simulink model "AD_SOAR_c7_V2f_c73_Clean_original"  (R2021a)
settings: Solver=ode4  StartTime=0.0  StopTime=TMax  FixedStep=Control.DT  RelTol=1e-3
undefined symbols (not defined in the file): Control, DiscIntNeverNeededParam, dLPF_slow, Downratelimiter, DT, IPCDQ_LPF, LPF_SetSmooth, OLControlParams, OutList, Parameters, PitchControlParams, rpm2radps, S_LowBPLim, Simulation, strmatch, TorqueControlParams, Upratelimiter
libraries: cstblocks x11, simulink x4, simulink_extras x1
(part 2 of 2)

== matlab function AD_SOAR_c7_V2f_c73_Clean_original/Baseline Controller/Wind Speed Estimator/MATLAB Function ==
  data: omega_g input; tau_g input; beta input; WE_params input; A_op input; vh output; xh input; P input; K input; xh output; P output; K output; dt input; Cx parameter; Debug output
function [vh,xh,P,K,Debug] = WSE_EKF(omega_g, tau_g, beta, WE_params, A_op, xh,P,K,dt, Cx)
% This function defines a WSE based off of an Extended Kalman Filter
% Inputs:
% Outputs:
% Nikhar Abbas

% Load R variables
J           = WE_params(1);             % Rotor Inertia
rho         = WE_params(2);             % Air density
Rr          = WE_params(3);             % Rotor Radius, R
Ng          = WE_params(4);             % Gearbox Ratio
ConeAngle   = WE_params(5);                % Cone Angle deg
ShaftTilt   = WE_params(6);                % Shaft Tilt deg

% Constants
H       = [1 0 0];
R       = 0.05;
L       = 4 * Rr;
Ti      = 0.2;

% MANDAR EDIT
% A       = pi*Rr^2;   % Rotor Swept Area, m^2 % ORIGINAL
A       = ( pi * ( Rr*cosd(ConeAngle) )^2 * cosd(ShaftTilt) ); % Projected Rotor Swept Area, m^2

% organize Inputs
om_r    = xh(1);
v_t     = xh(2);
v_m     = xh(3);
om_m    = omega_g  / Ng;

% Find current estimated operating conditions, and saturate
v_r     = v_t + v_m;
% MANDAR EDIT
% lambda  = om_r * Rr / v_r; % ORIGINAL
lambda  = om_r * Rr * cosd(ConeAngle) / v_r;
lambda  = max( min(lambda, Cx.TSR(end)), Cx.TSR(1));


% A_op (system pole) interpolation
% A_op    = interp1(R.WE_FOPoles_v,R.WE_FOPoles,xh(1) + xh(2));


% Cp interpolation
Cp      = interp2(Cx.BlPitch* pi/180, Cx.TSR, Cx.Cpmat, beta, lambda);
Cp      = max(0,Cp);


% Calculate Jacobians
F       = zeros(3,3);

F(1,1)      = A_op;
F(1,2)      = 1/(2*J)*rho*A*Cp*3*(v_m+v_t)^2*1/om_r;
F(1,3)      = 1/(2*J)*rho*A*Cp*3*(v_m+v_t)^2*1/om_r;

F(2,2)      = pi * v_m / (2*L);
F(2,3)      = pi * v_t / (2*L);  % this was 0


% Calculate Covariance
Q           = zeros(3,3);
Q(1,1)      = 1e-5;                     %in DZ WSE, 1e-6
Q(2,2)      = pi * v_m^3 * Ti^2 / L;
Q(3,3)      = 2^2/600;


%% Prediction Update

% states
tau_r       = 1/2 * rho * A * Cp * v_r^3 / om_r;       % Torque calculation
a           = pi * v_m / (2 * L);                           % Wind variance
dom_r       = 1/J * (tau_r - Ng * tau_g);
dv_t        = -a*v_t;
dv_m        = 0;
dxh         = [dom_r; dv_t; dv_m];

% forward euler
xh          = xh + dt*dxh;

% covariance
dP          = F*P + P*F' + Q - K*R*K';
P           = P + dt*dP;

% kalman gain
S           = H*P*H' + R;
K           = P * H' / S(1,1);   %DZ: this is odd, keep an eye on
% K           = P * H' * inv(S);   %DZ: this is odd, keep an eye on...was probably giving NJA stability issues

% output residual & update
y_til       = om_m - om_r;
xh          = xh + K*y_til;
P           = (eye(3) - K * H) * P;         % DZ: this is also different, but I think I've seen this form before


% Output Wind Speed Estimate
vh = v_m + v_t;

% Set Debug Outputs
Debug = Cp;

end

== matlab function AD_SOAR_c7_V2f_c73_Clean_original/Baseline Controller/Yaw Controller/ Yaw Control ==
  data: yawposeCommand output; time input; yawinc input; YAWCW input; YAWCCW input; YAWBRAKEYAW input; YawPos input; Yaw_status input; YawRate input; WINDSPEED input; WindDir input; yawinco output; YAWCWo output; YAWCCWo output; YAWBRAKEYAWo output; Yaw_statuso output; YAWERROR output
function [ yawposeCommand,yawinco,YAWCWo,YAWCCWo,YAWBRAKEYAWo,Yaw_statuso,YAWERROR]= Yaw(time,yawinc ,YAWCW,YAWCCW,YAWBRAKEYAW,YawPos,Yaw_status,YawRate,WINDSPEED, WindDir)
YAWERROR=(WindDir-YawPos*pi/180);
% yawinccheck=Simulation.DT*60000; 
yawinccheck=0.0125;%*60000;
%% Check if are currently yawing
if YAWCW~=0 || YAWCCW~=0    %Yawing already
    
    %%check that we've reached our destination
    if YAWCW && YawPos> yawinc || YAWCCW && YawPos< yawinc
        YAWCWo=0;
        YAWCCWo=0;
        yawinco=0;
        YAWBRAKEYAWo=0;
        yawposeCommand=0; % need to check
        Yaw_statuso=0;
        %YAWERROR_SV=YAWERROR_FV; ????
        %YAWERROR=YAWERROR;%?
        
    else
        YAWCWo=YAWCW;
        YAWCCWo=YAWCCW;
        yawinco=yawinc;%check
        yawposeCommand= yawinc;%YAWERROR+YawPos; % need to check
        YAWBRAKEYAWo=1;% need to check
        Yaw_statuso=1;
        
    end
    
    
    
    
    
%% Check if not currenlty yawing ,accumulate yaw error in  yawinc
 
else

    
    YAWCWo  = YAWCW ;
    YAWCCWo = YAWCCW ;
    yawinco = yawinc ;% need to check
    yawposeCommand = yawinc ; % need to check
    YAWBRAKEYAWo=YAWBRAKEYAW;
    Yaw_statuso = Yaw_status ;   
    
    
    
    
       if  abs(WINDSPEED)>4.0 && Yaw_status==0 && YAWBRAKEYAW == 0
                                                                                           
                if YAWERROR < 0
                    yawinco=yawinc-YAWERROR^2;
%                     YAWCWo=0;
%                     YAWCCWo=0;
%                     YAWBRAKEYAWo=0;
%                     yawposeCommand=yawinc-YAWERROR^2; % need to check
%                     Yaw_statuso=0;
                else
                    yawinco=yawinc+YAWERROR^2;
%                     YAWCWo=0;
%                     YAWCCWo=0;
%                     YAWBRAKEYAWo=0;
%                     yawposeCommand=yawinc-YAWERROR^2; % need to check
%                     Yaw_statuso=0;
                end
      end 
     if  abs( WINDSPEED )<1 && Yaw_status==0 &&YAWBRAKEYAW  == 0
            yawinco = 0;
            YAWCWo=0;
            YAWCCWo=0;
             YAWBRAKEYAWo=0;
            yawposeCommand=0; 
            Yaw_statuso=0;

     end
%         else 
%              
%            yawinco = yawinc; 
%            YAWCWo=YAWCW;
%            YAWCCWo=YAWCCW;
%            YAWBRAKEYAWo=YAWBRAKEYAW;
%            yawposeCommand=yawinc; % need to check
% %            Yaw_statuso=0;
%      end  
      
    
 %%If yawinc exceeds certain limits, decide to start yawing
      
     if yawinc > yawinccheck || yawinc <-1 * yawinccheck  %10 degree error for 10 minutes
%         yawposeCommand = YawPos + yawinc_temp;
        Yaw_statuso =1;
        YAWBRAKEYAWo= 1;
        yawinco=YawPos-YAWERROR;
        YAWCWo=1;
        YAWCCWo=1;
        yawposeCommand=YawPos-YAWERROR; % need to check
                   
%       if (YAWBRAKEPRESS < 500)  %wait until Pressure is under 500 to %       %delay can be used 
%       start yawing 
%       pause(2.0)
%      yawinc=YAWPOS-YAWERROR;


                        if     yawinc <= YawPos %Yaw CCW
                                YAWCWo  = 0 ;
                                YAWCCWo = 1 ;

                            else                 %Yaw CW
                                YAWCWo  = 1;
                                YAWCCWo = 0;
                        end


     end
      
     

    
    
end 
    
 
    
    
%     YAWCWo  = YAWCW ;
%     YAWCCWo = YAWCCW ;
%     yawinco = yawinc ;% need to check
%     yawposeCommand = yawinc ; % need to check
%     Yaw_statuso = Yaw_status ;
    
end

== matlab function AD_SOAR_c7_V2f_c73_Clean_original/Baseline Controller/PID Pitch controller/Variable Saturator1 ==
  data: pitchCommand input; lowerLimit input; pitchCommandOut output; upperLimit input; atLimit output
function [pitchCommandOut,atLimit] = variableSat(pitchCommand,lowerLimit,upperLimit)
%#codegen

if pitchCommand < lowerLimit
    pitchCommandOut = lowerLimit;
    atLimit          = 1;
    
elseif pitchCommand > upperLimit
    pitchCommandOut = upperLimit;
    atLimit         = 1;
    
else
    pitchCommandOut = pitchCommand;
    atLimit         = 0;
end

== matlab function AD_SOAR_c7_V2f_c73_Clean_original/Baseline Controller/Wind Speed Estimator/Soft Start ==
  data: startTime input; out output; endTime input; time input; generic input; actual input
function out = softStart(startTime,endTime,time,generic,actual)

as  = Af_sigma(startTime,endTime);
T   = [time^3,time^2,time,1]';

if time < startTime
    act = 0;
    gen = 1;
elseif time >= startTime && time < endTime
    act = as * T; 
    gen = 1 - as * T;
else
    act = 1;
    gen = 0;
end

out = act*actual + gen*generic;

== matlab function AD_SOAR_c7_V2f_c73_Clean_original/Baseline Controller/Cyclic Pitch controller/1P Cyclic Pitch Controller1/Lead Correction ==
  data: bdq input; b_cos output size=1; psi_o input; b_sin output size=1
function [b_cos,b_sin] = fcn(bdq, psi_o)
% This block supports the Embedded MATLAB subset.
% See the help menu for details. 

b_cos=[cosd(psi_o) sind(psi_o)]*bdq;
b_sin=[-sind(psi_o) cosd(psi_o)]*bdq;

== matlab function AD_SOAR_c7_V2f_c73_Clean_original/Baseline Controller/Cyclic Pitch controller/1P Cyclic Pitch Controller1/d-q transformation ==
  data: RootMyb input; M_tilt output; Az input; M_yaw output; NumBl input
function [M_tilt,M_yaw] = fwdMBC2(RootMyb, Az, NumBl)
% This block supports the Embedded MATLAB subset.
% See the help menu for details.

if NumBl == 2
    
    My=RootMyb-mean(RootMyb(1:2)); %remove mean
    
    M_tilt = [cosd(Az) cosd(Az+180) 0]*My;
    M_yaw =  [sind(Az) sind(Az+180) 0]*My;
else
%     My=RootMyb-mean(RootMyb); %remove mean
    My=RootMyb;
    M_tilt = (2/3).*[cosd(Az) cosd(Az+120) cosd(Az+240)]*My;
    M_yaw =  (2/3).*[sind(Az) sind(Az+120) sind(Az+240)]*My;
end

== matlab function AD_SOAR_c7_V2f_c73_Clean_original/Baseline Controller/Cyclic Pitch controller/1P Cyclic Pitch Controller1/inverse d-q transformation ==
  data: bdq input; b1 output size=1; Az input; b2 output size=1; NumBl input; b3 output size=1
function [b1,b2,b3] = bckMBC2(bdq, Az, NumBl)
% This block supports the Embedded MATLAB subset.
% See the help menu for details.


if NumBl == 2
    
    b1=[cosd(Az) sind(Az)]*bdq;
    b2=[cosd(Az - 180) sind(Az - 180)]*bdq;
    b3=0;
    
else
    b1=[cosd(Az) sind(Az)]*bdq;
    b2=[cosd(Az + 120) sind(Az + 120)]*bdq;
    b3=[cosd(Az + 240) sind(Az + 240)]*bdq;
    
end

== matlab function AD_SOAR_c7_V2f_c73_Clean_original/Baseline Controller/Cyclic Pitch controller/1P Cyclic Pitch Controller1/saturation (limit schedule)1 ==
  data: bdq_unsat input size=[2 1]; bdq output; b_avg input; M0 input; PitchControlParams parameter; k output
%limit b_d and b_q so b_1,2,or3 does not get bigger than b_avg (the sinusoids don't get cut off at zero)
%unless b_avg is <0, then limit to 0
%at_limit is 1 if limited, 0 otherwise

function [bdq,k]  = fcn(bdq_unsat, b_avg, M0,PitchControlParams)

MODE    = PitchControlParams.IPCDQ_MODE;  % 1 no IPC below rated (no power loss), 2 IPC always on, 3
M0_set  = PitchControlParams.IPCDQ_M0_set;
k_sat   = PitchControlParams.IPCDQ_k_sat;

if MODE == 1
    
    if (b_avg <=deg2rad(PitchControlParams.theta_fine + 1))
        bdq=[0;0];
        k = 0;
    else
        if (norm(bdq_unsat,2) <= b_avg)
            bdq = bdq_unsat;
            k = 1;
        else
            bdq=bdq_unsat*(b_avg/norm(bdq_unsat,2));
            k = (b_avg/norm(bdq_unsat,2));
        end
    end
elseif MODE == 2
    %     if (b_avg <= deg2rad(PitchControlParams.theta_fine+0.05))
    %         bdq=[0;0];
    %         k = 0;
    %     else
    if (norm(bdq_unsat,2) > deg2rad(15))
        bdq = bdq_unsat*(deg2rad(15)/norm(bdq_unsat,2));
        k = (deg2rad(15)/norm(bdq_unsat,2));
    else
        bdq = bdq_unsat;
        k = 1;
    end
    %     end
else  % MODE 3
    if (M0 > M0_set - 1/(2*k_sat))
        if (M0 > M0_set + 1/(2*k_sat))
            bdq = bdq_unsat;
            k = 1;
        else
            k = k_sat*(M0-M0_set)+1/2;
            bdq = k*bdq_unsat;
        end
    else
        bdq = [0;0];
        k = 0;
    end
end
%
% if (b_avg <=0)
%         bdq = bdq_unsat;
% else
%     if (norm(bdq_unsat,2) <= b_avg)
%         bdq = bdq_unsat;
%     else
%         bdq = bdq_unsat;
%     end
% end

== matlab function AD_SOAR_c7_V2f_c73_Clean_original/Baseline Controller/Torque Controller/LUT-Based Torque Control/Baseline Torque Cotnroller ==
  settings: updateMethod=DISCRETE  sampleTime=Control.DT
  data: W_hss input; Pitch input; genTorque output; region output; S_LowBPLim input; TorqueControlParams parameter
function [genTorque, region] = regionSelectTq_Flex( W_hss, Pitch, S_LowBPLim, TorqueControlParams)
% This block supports an embeddable subset of the MATLAB language.
% See the help menu for details.


%% Assign Constants

wg_rated    = TorqueControlParams.wg_rated;
T_rated     = TorqueControlParams.T_rated;
w2_high     = TorqueControlParams.w2_high;
w1_high     = TorqueControlParams.w1_high;
wg_min      = TorqueControlParams.wg_min;
m2_5        = TorqueControlParams.m2_5;
c2_5        = TorqueControlParams.c2_5;
m1_5        = TorqueControlParams.m1_5;
c1_5        = TorqueControlParams.c1_5;
k_opt       = TorqueControlParams.k_opt;


%% Switch based on Gen. Speed

if (((S_LowBPLim==0)&&(W_hss >= wg_rated)) || ((S_LowBPLim==1)&&((Pitch >= TorqueControlParams.fine_pitch+3) || (W_hss >= wg_rated)))) %Region 3 calcs
    region=3;
    genTorque = T_rated;

elseif (W_hss >= w2_high)                %Region 2.5
    region=2.5;    
%     genTorque = m2_5 * W_hss + c2_5;
    genTorque = k_opt * W_hss^2; % MANDAR TEST
elseif (W_hss >= w1_high)                    %Region 2
    region=2;
    genTorque = k_opt * W_hss^2;
    
elseif (W_hss > wg_min)                    %Region 1.5
    region=1.5;
        genTorque = m1_5 * W_hss + c1_5;
%     genTorque = k_opt * W_hss^2; % MANDAR TEST
else                                    %Region 1
    region=1;
    genTorque = 0;
end

% if startup
%     region=1;
%     genTorque = 0;
% end
